simulink model "RemoteCHIL"  (Simulink 8.1)
settings: Solver=ode1  StartTime=0.0  StopTime=inf  FixedStep=Ts  MaxStep=1e-3  RelTol=1e-3
PostLoadFcn:
  | NREL_Mode=3; BANSHEE_init;
InitFcn:
  | NREL_Mode=3; BANSHEE_init;
values from neighbouring files (symbols this model uses):
  F4 = xlsread('F4_relay_nrel.xlsx')    [relay_settings_init.m]
  Ts = 100E-6    (= 0.0001)    [BANSHEE_init.m]    (also in Ghost_init.m)
undefined symbols (not defined in the file or in its folder): Left, Stim, type, V
libraries: simulink x50, relay_modbus_lib x11, simulink_extras x10, rtio_generic_modbus x6, rtlab x5, RMS_lib x4, cables_lib x3, relay_PLL_lib x3, PHIL_lib x2, breaker_lib x2, powerlib_extras x2, relay_ANSI_functions_lib x2
(part 3 of 3)

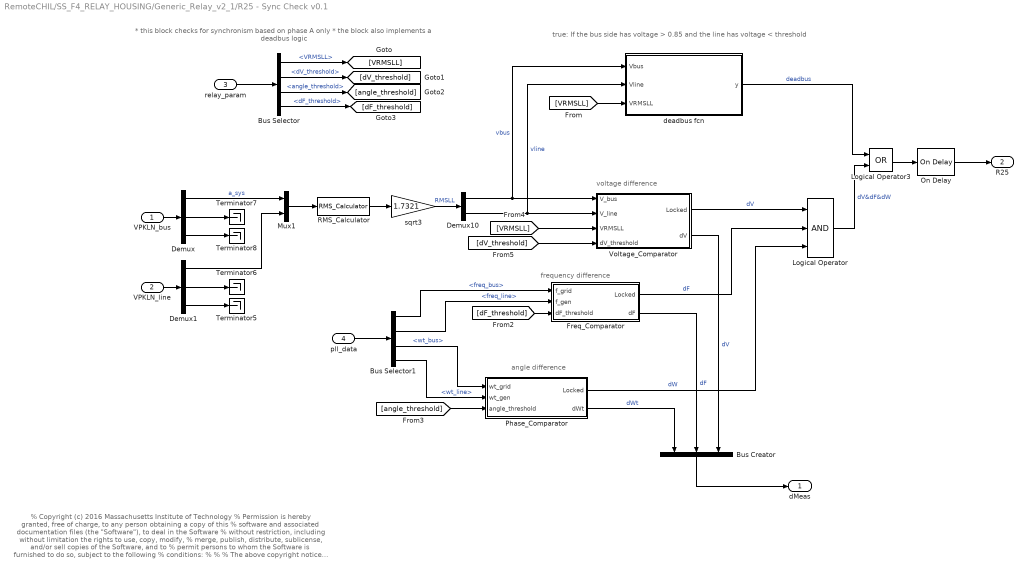
== system RemoteCHIL/SS_F4_RELAY_HOUSING/Generic_Relay_v2_1/R25 - Sync Check v0.1 ==
  note: * this block checks for synchronism based on phase A only
      | * the block also implements a deadbus logic
  note: angle difference
  note: frequency difference
  note: voltage difference
  note: true: If the bus side has voltage > 0.85 and the line has voltage < threshold
  note: % Copyright (c) 2016 Massachusetts Institute of Technology
      | % Permission is hereby granted, free of charge, to any person obtaining a copy of this
      | % software and associated documentation files (the "Software"), to deal in the Software
      | % without restriction, including without limitation the rights to use, copy, modify,
      | % merge, publish, distribute, sublicense, and/or sell copies of the Software, and to
      | % permit persons to whom the Software is furnished to do so, subject to the following
      | % conditions:
      | %
      | %
      | % The above copyright notice and this permission notice shall be included in
      | % all copies or substantial portions of the Software.
      | %
      | % THE SOFTWARE IS PROVIDED "AS IS", WITHOUT WARRANTY OF ANY KIND, EXPRESS OR IMPLIED,
      | % INCLUDING BUT NOT LIMITED TO THE WARRANTIES OF MERCHANTABILITY, FITNESS FOR A
      | % PARTICULAR PURPOSE AND NONINFRINGEMENT. IN NO EVENT SHALL THE AUTHORS OR COPYRIGHT
      | % HOLDERS BE LIABLE FOR ANY CLAIM, DAMAGES OR OTHER LIABILITY, WHETHER IN AN ACTION
      | % OF CONTRACT, TORT OR OTHERWISE, ARISING FROM, OUT OF OR IN CONNECTION WITH THE
      | % SOFTWARE OR THE USE OR OTHER DEALINGS IN THE SOFTWARE.
      | %
      | %
      | %%
  VPKLN_bus : Inport
  VPKLN_line : Inport  Port=2
  relay_param : Inport  Port=3
  pll_data : Inport  Port=4
  Bus Creator : BusCreator  Inputs=3
  Bus Selector : BusSelector  OutputSignals=VRMSLL,dV_threshold,angle_threshold,dF_threshold
  Bus Selector1 : BusSelector  OutputSignals=freq_bus,freq_line,wt_bus,wt_line
  Demux : Demux  Outputs=3
  Demux1 : Demux  Outputs=3
  Demux10 : Demux  Outputs=2
  Freq_Comparator : Subsystem
  Logical Operator : Logic  Inputs=3  AllPortsSameDT=off  OutDataTypeStr=boolean
  Logical Operator3 : Logic  Operator=OR  AllPortsSameDT=off  OutDataTypeStr=boolean
  Mux1 : Mux  Inputs=2
  On Delay : powerlib_meascontrol/Logic/On Delay  DelayType=On delay  delay=0.05  ic=0  Ts=Ts
  Phase_Comparator : Subsystem
  RMS_Calculator : RMS_lib/RMS_Calculator  Ts=Ts
  Terminator{5..8} (4 alike) : Terminator
  Voltage_Comparator : Subsystem
  deadbus fcn : MATLAB Function  TreatAsAtomicUnit=on
  sqrt3 : Gain  Gain=1.7321
  dMeas : Outport
  R25 : Outport  Port=2
  wires:
  Bus Creator/1 -> dMeas/1
  Phase_Comparator/2(dWt) -> Bus Creator/1  "dWt"
  Freq_Comparator/2(dF) -> Bus Creator/2  "dF"
  Voltage_Comparator/2(dV) -> Bus Creator/3  "dV"
  [dV_threshold] -> Voltage_Comparator/4(dV_threshold)
  [VRMSLL] -> Voltage_Comparator/3(VRMSLL)
  [angle_threshold] -> Phase_Comparator/3(angle_threshold)
  [dF_threshold] -> Freq_Comparator/3(dF_threshold)
  Bus Selector/4 -> [dF_threshold]  "<dF_threshold>"
  Bus Selector/3 -> [angle_threshold]  "<angle_threshold>"
  Bus Selector/2 -> [dV_threshold]  "<dV_threshold>"
  Bus Selector/1 -> [VRMSLL]  "<VRMSLL>"
  relay_param/1 -> Bus Selector/1
  [VRMSLL] -> deadbus fcn/3(VRMSLL)
  sqrt3/1 -> Demux10/1  "RMSLL"
  Mux1/1 -> RMS_Calculator/1
  RMS_Calculator/1 -> sqrt3/1
  Phase_Comparator/1(Locked) -> Logical Operator/3  "dW"
  Freq_Comparator/1(Locked) -> Logical Operator/2  "dF"
  Voltage_Comparator/1(Locked) -> Logical Operator/1  "dV"
  Demux10/2 -> deadbus fcn/2(Vline), Voltage_Comparator/2(V_line)  "vline"
  Bus Selector1/4 -> Phase_Comparator/2(wt_gen)  "<wt_line>"
  Bus Selector1/3 -> Phase_Comparator/1(wt_grid)  "<wt_bus>"
  Bus Selector1/2 -> Freq_Comparator/2(f_gen)  "<freq_line>"
  Bus Selector1/1 -> Freq_Comparator/1(f_grid)  "<freq_bus>"
  Demux10/1 -> deadbus fcn/1(Vbus), Voltage_Comparator/1(V_bus)  "vbus"
  Demux/1 -> Mux1/1  "a_sys"
  Demux1/1 -> Mux1/2
  Demux1/2 -> Terminator6/1
  Demux1/3 -> Terminator5/1
  Demux/2 -> Terminator7/1
  Demux/3 -> Terminator8/1
  VPKLN_bus/1 -> Demux/1
  VPKLN_line/1 -> Demux1/1
  deadbus fcn/1(y) -> Logical Operator3/1  "deadbus"
  Logical Operator/1 -> Logical Operator3/2  "dV&dF&dW"
  pll_data/1 -> Bus Selector1/1
  Logical Operator3/1 -> On Delay/1
  On Delay/1 -> R25/1

== system RemoteCHIL/SS_F4_RELAY_HOUSING/Generic_Relay_v2_1/bitwise_faults ==
  note: Constant array has LSB on most left.
  S : Inport
  Bitwise Operator : simulink/Logic and Bit Operations/Bitwise Operator  logicop=OR  UseBitMask=off  NumInputPorts=16  BitMask=bin2dec('11011001')  BitMaskRealWorld=Stored Integer
  Data Type Conversion : DataTypeConversion  OutDataTypeStr=uint16
  Data Type Conversion1 : DataTypeConversion  OutDataTypeStr=double
  Demux : Demux  Outputs=16
  Shift Arithmetic : ArithShift  BitShiftNumber=1  BitShiftDirection=Left
  Shift Arithmetic1 : ArithShift  BitShiftNumber=2  BitShiftDirection=Left
  Shift Arithmetic10 : ArithShift  BitShiftNumber=11  BitShiftDirection=Left
  Shift Arithmetic11 : ArithShift  BitShiftNumber=12  BitShiftDirection=Left
  Shift Arithmetic12 : ArithShift  BitShiftNumber=13  BitShiftDirection=Left
  Shift Arithmetic13 : ArithShift  BitShiftNumber=14  BitShiftDirection=Left
  Shift Arithmetic14 : ArithShift  BitShiftNumber=15  BitShiftDirection=Left
  Shift Arithmetic2 : ArithShift  BitShiftNumber=3  BitShiftDirection=Left
  Shift Arithmetic3 : ArithShift  BitShiftNumber=4  BitShiftDirection=Left
  Shift Arithmetic4 : ArithShift  BitShiftNumber=5  BitShiftDirection=Left
  Shift Arithmetic5 : ArithShift  BitShiftNumber=6  BitShiftDirection=Left
  Shift Arithmetic6 : ArithShift  BitShiftNumber=7  BitShiftDirection=Left
  Shift Arithmetic7 : ArithShift  BitShiftNumber=8  BitShiftDirection=Left
  Shift Arithmetic8 : ArithShift  BitShiftNumber=9  BitShiftDirection=Left
  Shift Arithmetic9 : ArithShift  BitShiftNumber=10  BitShiftDirection=Left
  s : Outport
  wires:
  Data Type Conversion/1 -> Demux/1
  S/1 -> Data Type Conversion/1
  Bitwise Operator/1 -> Data Type Conversion1/1
  Data Type Conversion1/1 -> s/1
  Demux/1 -> Bitwise Operator/1
  Demux/2 -> Shift Arithmetic/1
  Demux/3 -> Shift Arithmetic1/1
  Demux/4 -> Shift Arithmetic2/1
  Demux/5 -> Shift Arithmetic3/1
  Demux/6 -> Shift Arithmetic4/1
  Demux/7 -> Shift Arithmetic5/1
  Shift Arithmetic/1 -> Bitwise Operator/2
  Shift Arithmetic1/1 -> Bitwise Operator/3
  Shift Arithmetic2/1 -> Bitwise Operator/4
  Shift Arithmetic3/1 -> Bitwise Operator/5
  Shift Arithmetic4/1 -> Bitwise Operator/6
  Shift Arithmetic5/1 -> Bitwise Operator/7
  Shift Arithmetic9/1 -> Bitwise Operator/11
  Shift Arithmetic6/1 -> Bitwise Operator/8
  Shift Arithmetic8/1 -> Bitwise Operator/10
  Shift Arithmetic7/1 -> Bitwise Operator/9
  Demux/8 -> Shift Arithmetic6/1
  Demux/9 -> Shift Arithmetic7/1
  Demux/10 -> Shift Arithmetic8/1
  Demux/11 -> Shift Arithmetic9/1
  Demux/12 -> Shift Arithmetic10/1
  Demux/13 -> Shift Arithmetic11/1
  Demux/14 -> Shift Arithmetic12/1
  Demux/15 -> Shift Arithmetic13/1
  Demux/16 -> Shift Arithmetic14/1
  Shift Arithmetic10/1 -> Bitwise Operator/12
  Shift Arithmetic11/1 -> Bitwise Operator/13
  Shift Arithmetic12/1 -> Bitwise Operator/14
  Shift Arithmetic13/1 -> Bitwise Operator/15
  Shift Arithmetic14/1 -> Bitwise Operator/16

== system RemoteCHIL/SS_F4_RELAY_HOUSING/Generic_Relay_v2_1/dfdt ==
  note: Hz/s
  note: Hz
  freq : Inport
  Delay1 : Delay  DelayLength=3/60/(Ts)  UseCircularBuffer=on
  Gain : Gain  Gain=60/3
  Sum3 : Sum  Inputs=|-+
  dfdt : Outport
  wires:
  freq/1 -> Sum3/2, Delay1/1
  Sum3/1 -> Gain/1  "df"
  Delay1/1 -> Sum3/1
  Gain/1 -> dfdt/1  "dfdt"

== system RemoteCHIL/SS_F4_RELAY_HOUSING/Generic_Relay_v2_1/pf bitwise ==
  note: Constant array has LSB on most left.
  S : Inport
  Bitwise Operator : simulink/Logic and Bit Operations/Bitwise Operator  logicop=OR  UseBitMask=off  NumInputPorts=2  BitMask=bin2dec('11011001')  BitMaskRealWorld=Stored Integer
  Data Type Conversion : DataTypeConversion  OutDataTypeStr=uint16
  Data Type Conversion1 : DataTypeConversion  OutDataTypeStr=double
  Demux : Demux  Outputs=2
  Shift Arithmetic : ArithShift  BitShiftNumber=1  BitShiftDirection=Left
  s : Outport
  wires:
  Shift Arithmetic/1 -> Bitwise Operator/2
  Demux/2 -> Shift Arithmetic/1
  Demux/1 -> Bitwise Operator/1
  Data Type Conversion1/1 -> s/1
  Bitwise Operator/1 -> Data Type Conversion1/1
  S/1 -> Data Type Conversion/1
  Data Type Conversion/1 -> Demux/1

== system RemoteCHIL/SS_F4_RELAY_HOUSING/Misc_data/VRMSLL ==
  In1 : Inport
  Bus Selector29 : BusSelector  OutputSignals=zero,zero,zero,zero,zero,zero,F4.LOAD_DATA.F4_I7.VRMSLL,F4.LOAD_DATA.F4_I8.VRMSLL,zero,zero,zero,zero,zero,zero,F4.LOAD_DATA.F4_P7.VRMSLL,F4.LOAD_DATA.F4_P8.VRMSLL,zero,zero,zero,zero,zero,zero,F4.LOAD_DATA.F4_C7.VRMSLL,F4.LOAD_DATA.F4_C8.VRMSLL,F4.LOAD_DATA.F4_C9.VRMSLL
  Mux : Mux  Inputs=25
  Out1 : Outport
  wires:
  In1/1 -> Bus Selector29/1
  Mux/1 -> Out1/1
  Bus Selector29/1 -> Mux/1  "<zero>"
  Bus Selector29/25 -> Mux/25  "<VRMSLL>"
  Bus Selector29/24 -> Mux/24  "<VRMSLL>"
  Bus Selector29/17 -> Mux/17  "<zero>"
  Bus Selector29/18 -> Mux/18  "<zero>"
  Bus Selector29/19 -> Mux/19  "<zero>"
  Bus Selector29/20 -> Mux/20  "<zero>"
  Bus Selector29/21 -> Mux/21  "<zero>"
  Bus Selector29/22 -> Mux/22  "<zero>"
  Bus Selector29/23 -> Mux/23  "<VRMSLL>"
  Bus Selector29/10 -> Mux/10  "<zero>"
  Bus Selector29/11 -> Mux/11  "<zero>"
  Bus Selector29/12 -> Mux/12  "<zero>"
  Bus Selector29/13 -> Mux/13  "<zero>"
  Bus Selector29/14 -> Mux/14  "<zero>"
  Bus Selector29/15 -> Mux/15  "<VRMSLL>"
  Bus Selector29/16 -> Mux/16  "<VRMSLL>"
  Bus Selector29/3 -> Mux/3  "<zero>"
  Bus Selector29/4 -> Mux/4  "<zero>"
  Bus Selector29/5 -> Mux/5  "<zero>"
  Bus Selector29/6 -> Mux/6  "<zero>"
  Bus Selector29/7 -> Mux/7  "<VRMSLL>"
  Bus Selector29/8 -> Mux/8  "<VRMSLL>"
  Bus Selector29/9 -> Mux/9  "<zero>"
  Bus Selector29/2 -> Mux/2  "<zero>"

== system RemoteCHIL/SS_F4_RELAY_HOUSING/Misc_data/kW ==
  In1 : Inport
  Bus Selector28 : BusSelector  OutputSignals=zero,zero,zero,zero,zero,zero,F4.LOAD_DATA.F4_I7.kw,F4.LOAD_DATA.F4_I8.kw,zero,zero,zero,zero,zero,zero,F4.LOAD_DATA.F4_P7.kw,F4.LOAD_DATA.F4_P8.kw,zero,zero,zero,zero,zero,zero,F4.LOAD_DATA.F4_C7.kw,F4.LOAD_DATA.F4_C8.kw,F4.LOAD_DATA.F4_C9.kw
  Mux : Mux  Inputs=25
  Out1 : Outport
  wires:
  In1/1 -> Bus Selector28/1
  Mux/1 -> Out1/1
  Bus Selector28/25 -> Mux/25  "<kw>"
  Bus Selector28/24 -> Mux/24  "<kw>"
  Bus Selector28/23 -> Mux/23  "<kw>"
  Bus Selector28/22 -> Mux/22  "<zero>"
  Bus Selector28/21 -> Mux/21  "<zero>"
  Bus Selector28/20 -> Mux/20  "<zero>"
  Bus Selector28/19 -> Mux/19  "<zero>"
  Bus Selector28/18 -> Mux/18  "<zero>"
  Bus Selector28/17 -> Mux/17  "<zero>"
  Bus Selector28/16 -> Mux/16  "<kw>"
  Bus Selector28/15 -> Mux/15  "<kw>"
  Bus Selector28/14 -> Mux/14  "<zero>"
  Bus Selector28/13 -> Mux/13  "<zero>"
  Bus Selector28/12 -> Mux/12  "<zero>"
  Bus Selector28/11 -> Mux/11  "<zero>"
  Bus Selector28/10 -> Mux/10  "<zero>"
  Bus Selector28/9 -> Mux/9  "<zero>"
  Bus Selector28/8 -> Mux/8  "<kw>"
  Bus Selector28/7 -> Mux/7  "<kw>"
  Bus Selector28/6 -> Mux/6  "<zero>"
  Bus Selector28/5 -> Mux/5  "<zero>"
  Bus Selector28/4 -> Mux/4  "<zero>"
  Bus Selector28/3 -> Mux/3  "<zero>"
  Bus Selector28/2 -> Mux/2  "<zero>"
  Bus Selector28/1 -> Mux/1  "<zero>"

== system RemoteCHIL/SS_F4_RELAY_HOUSING/Relay_data/ExtractF4 ==
  In1 : Inport
  Bus Selector47 : BusSelector  OutputSignals=F4_CB_1,F4_CB_2,F4_CB_3,F4_CB_4,F4_CB_5,F4_CB_6
  Bus Selector{48..52,61} (6 alike) : BusSelector  OutputSignals=m.kw,m.kvar,m.Vpu,m.Hz,m.status  OutputAsBus=on
  Mux13 : Mux  Inputs=6
  Out1 : Outport
  wires:
  Bus Selector61/1 -> Mux13/3
  Bus Selector47/5 -> Bus Selector51/1  "<F4_CB_5>"
  Bus Selector49/1 -> Mux13/2
  Bus Selector47/2 -> Bus Selector49/1  "<F4_CB_2>"
  Bus Selector47/3 -> Bus Selector61/1  "<F4_CB_3>"
  Bus Selector47/6 -> Bus Selector52/1  "<F4_CB_6>"
  Bus Selector52/1 -> Mux13/6
  Mux13/1 -> Out1/1
  In1/1 -> Bus Selector47/1
  Bus Selector50/1 -> Mux13/4
  Bus Selector47/1 -> Bus Selector48/1  "<F4_CB_1>"
  Bus Selector47/4 -> Bus Selector50/1  "<F4_CB_4>"
  Bus Selector48/1 -> Mux13/1
  Bus Selector51/1 -> Mux13/5

== system RemoteCHIL/SS_F4_RELAY_HOUSING/Relay_data/Subsystem1 ==
  F4 : Inport
  Bus Selector1 : BusSelector  OutputSignals=CB_meas.relay_out.m.kw,CB_meas.relay_out.m.kvar,CB_meas.relay_out.m.Vpu,CB_meas.relay_out.m.Hz,CB_meas.cb_meas.Status  OutputAsBus=on
  Bus Selector10 : BusSelector  OutputSignals=m.kw,m.kvar,m.Vpu,m.Hz,m.status  OutputAsBus=on
  Bus Selector12 : BusSelector  OutputSignals=CB_meas.relay_out.m.kw,CB_meas.relay_out.m.kvar,CB_meas.relay_out.m.Vpu,CB_meas.relay_out.m.Hz,CB_meas.cb_meas.Status  OutputAsBus=on
  Bus Selector3 : BusSelector  OutputSignals=cb.relay_out
  Bus Selector9 : BusSelector  OutputSignals=GEN3_DATA,ESS_DATA,PV_DATA
  Constant{1..4} (4 alike) : Constant  Value=zeros(1,5)
  Mux : Mux  Inputs=7
  Out1 : Outport
  wires:
  Mux/1 -> Out1/1
  Constant2/1 -> Mux/4
  Constant1/1 -> Mux/2
  Constant3/1 -> Mux/1
  Constant4/1 -> Mux/3
  F4/1 -> Bus Selector9/1
  Bus Selector9/1 -> Bus Selector3/1  "<GEN3_DATA>"
  Bus Selector3/1 -> Bus Selector10/1  "<relay_out>"
  Bus Selector10/1 -> Mux/5
  Bus Selector12/1 -> Mux/6
  Bus Selector9/2 -> Bus Selector12/1  "<ESS_DATA>"
  Bus Selector1/1 -> Mux/7
  Bus Selector9/3 -> Bus Selector1/1  "<PV_DATA>"

== system RemoteCHIL/SS_F4_RELAY_HOUSING/Generic_Relay_v2_1/R25 - Sync Check v0.1/Freq_Comparator ==
  note: This block compares the frequency at the circuit breaker terminals
      | * if the difference is less than threshold dF_threshold, then outputs 1
  f_grid : Inport
  f_gen : Inport  Port=2
  dF_threshold : Inport  Port=3
  Fcn2 : Fcn  Expr=abs(u(2)-u(1)) <= u(3)
  Mux1 : Mux  Inputs=3
  Sum : Sum  Inputs=+-
  Locked : Outport
  dF : Outport  Port=2
  wires:
  Sum/1 -> dF/1
  f_grid/1 -> Mux1/1, Sum/2
  f_gen/1 -> Mux1/2, Sum/1
  dF_threshold/1 -> Mux1/3
  Fcn2/1 -> Locked/1
  Mux1/1 -> Fcn2/1

== system RemoteCHIL/SS_F4_RELAY_HOUSING/Generic_Relay_v2_1/R25 - Sync Check v0.1/Phase_Comparator ==
  note: This block compares the angle (phase A only) at the circuit breaker terminals
      | * if the difference is less than threshold angle_threshold, then outputs 1
  wt_grid : Inport
  wt_gen : Inport  Port=2
  angle_threshold : Inport  Port=3
  Abs : Abs
  Fcn1 : Fcn  Expr=u(1) <= u(2)  SampleTime=Ts
  Mux1 : Mux  Inputs=2
  Radians to Degrees : simulink_extras/Transformations/Radians to Degrees
  Sum1 : Sum  Inputs=|-+
  WrapPi : Subsystem
  Locked : Outport
  dWt : Outport  Port=2
  wires:
  WrapPi/1(Out1) -> Abs/1, dWt/1
  Sum1/1 -> WrapPi/1(In1)
  wt_grid/1 -> Sum1/1
  wt_gen/1 -> Sum1/2
  Radians to Degrees/1 -> Mux1/1  "R2D"
  Mux1/1 -> Fcn1/1
  angle_threshold/1 -> Mux1/2
  Fcn1/1 -> Locked/1  "bool"
  Abs/1 -> Radians to Degrees/1  "diff"

== system RemoteCHIL/SS_F4_RELAY_HOUSING/Generic_Relay_v2_1/R25 - Sync Check v0.1/Voltage_Comparator ==
  note: This block compares the voltage at the circuit breaker terminals
      | * if the difference is less than threshold, then outputs 1
  note: dV_threshold% of the nominal VRMSLL
  V_bus : Inport
  V_line : Inport  Port=2
  VRMSLL : Inport  Port=3
  dV_threshold : Inport  Port=4
  Abs : Abs
  Constant : Constant  Value=0.6
  Logical Operator : Logic  AllPortsSameDT=off  OutDataTypeStr=boolean
  Product : Product
  Product1 : Product
  Relational Operator : RelationalOperator  Operator=<=  OutDataTypeStr=boolean
  Relational Operator1 : RelationalOperator  OutDataTypeStr=boolean
  Sum : Sum  Inputs=+-
  a : Gain  Gain=0.01
  Locked : Outport
  dV : Outport  Port=2
  wires:
  Sum/1 -> dV/1, Abs/1
  Product/1 -> Relational Operator/2
  VRMSLL/1 -> Product1/1, Product/1
  dV_threshold/1 -> a/1  "[%]"
  V_bus/1 -> Relational Operator1/1, Sum/2
  V_line/1 -> Sum/1
  Relational Operator/1 -> Logical Operator/1  "thshld"
  a/1 -> Product/2  "[dec]"
  Logical Operator/1 -> Locked/1
  Constant/1 -> Product1/2
  Product1/1 -> Relational Operator1/2
  Abs/1 -> Relational Operator/1
  Relational Operator1/1 -> Logical Operator/2

== system RemoteCHIL/SS_F4_RELAY_HOUSING/Generic_Relay_v2_1/R25 - Sync Check v0.1/Phase_Comparator/WrapPi ==
  In1 : Inport
  Compare To Constant1 : simulink/Logic and Bit Operations/Compare To Constant  relop=<=  const=-pi  OutDataTypeStr=boolean
  Compare To Constant2 : simulink/Logic and Bit Operations/Compare To Constant  relop=>=  const=pi  OutDataTypeStr=boolean
  Gain1 : Gain  Gain=2*pi
  Gain2 : Gain  Gain=2*pi
  Sum : Sum  Inputs=++-
  Out1 : Outport
  wires:
  Compare To Constant2/1 -> Gain2/1
  Compare To Constant1/1 -> Gain1/1
  In1/1 -> Sum/2, Compare To Constant1/1, Compare To Constant2/1
  Gain2/1 -> Sum/3
  Gain1/1 -> Sum/1
  Sum/1 -> Out1/1

== matlab function SS_F4_RELAY_HOUSING/Generic_Relay_v2_1/R25 - Sync Check v0.1/deadbus fcn ==
  data: Vbus input double; y output double; Vline input double; VRMSLL input double
% Copyright (c) 2016 Massachusetts Institute of Technology
% Permission is hereby granted, free of charge, to any person obtaining a copy of this
% software and associated documentation files (the "Software"), to deal in the Software
% without restriction, including without limitation the rights to use, copy, modify,
% merge, publish, distribute, sublicense, and/or sell copies of the Software, and to
% permit persons to whom the Software is furnished to do so, subject to the following
% conditions:
%
%
% The above copyright notice and this permission notice shall be included in
% all copies or substantial portions of the Software.
%
% THE SOFTWARE IS PROVIDED "AS IS", WITHOUT WARRANTY OF ANY KIND, EXPRESS OR IMPLIED,
% INCLUDING BUT NOT LIMITED TO THE WARRANTIES OF MERCHANTABILITY, FITNESS FOR A
% PARTICULAR PURPOSE AND NONINFRINGEMENT. IN NO EVENT SHALL THE AUTHORS OR COPYRIGHT
% HOLDERS BE LIABLE FOR ANY CLAIM, DAMAGES OR OTHER LIABILITY, WHETHER IN AN ACTION
% OF CONTRACT, TORT OR OTHERWISE, ARISING FROM, OUT OF OR IN CONNECTION WITH THE
% SOFTWARE OR THE USE OR OTHER DEALINGS IN THE SOFTWARE.
%
%
%%

function y = fcn(Vbus, Vline, VRMSLL)
%#codegen
if isnan(Vbus)
    Vbus=0;
elseif isnan(Vline)
    Vline = 0;
end

% voltage threshold for deadbus
if VRMSLL > 520
    threshold = VRMSLL * 0.03; % @ 3%
else
    threshold = VRMSLL * 0.05; % @ 5%
end

% selecting 10V as the deadbus band - similar to SEL751
% threshold = 10;

% bounding open-circuit voltage at 120%
a = (Vbus>(VRMSLL*0.85)) && (Vbus<(VRMSLL*1.20)) && (Vline < threshold);
%b = (Vline>(VRMSLL*0.8)) && (Vline<(VRMSLL*1.20)) && (Vbus < threshold); -
% disabled for CB401 - voltage must be available on grid sim
% c = (Vline < threshold) && (Vbus < threshold);
y = a; %||b||c;
